simulink model "simulink_problem_2_9_98_14"  (R2014a)
settings: Solver=ode45  SolverMode=SingleTasking  StartTime=0.0  StopTime=10.0  RelTol=1e-3
settings Model: CovMetricSettings=dwe  CovHtmlReporting=off  covSaveCumulativeToWorkspaceVar=off  CovSaveSingleToWorkspaceVar=off  CovExternalEMLEnable=on  CovSFcnEnable=on  Creator=ghost  LastModifiedBy=ghost
settings DataIOCC: LimitDataPoints=off  SaveFormat=StructureWithTime
settings DebuggingCC: MergeDetectMultiDrivingBlocksExec=error  SolverPrmCheckMsg=none  FrameProcessingCompatibilityMsg=error  SFUnexpectedBacktrackingDiag=error  SFNoUnconditionalDefaultTransitionDiag=error
settings HardwareCC: ProdBitPerPointer=64  ProdLargestAtomicFloat=Float  ProdIntDivRoundTo=Zero  ProdEndianess=LittleEndian  ProdHWDeviceType=Specified
settings ModelReferenceCC: PropagateSignalLabelsOutOfModel=on
settings GRTTargetCC: TargetLangStandard=C99 (ISO)  GeneratePreprocessorConditionals=Use local settings

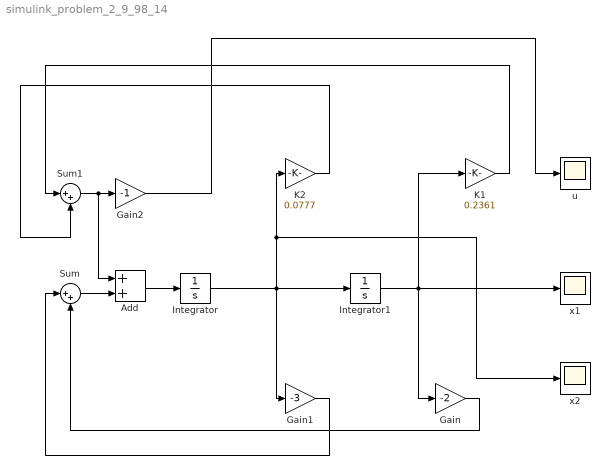
== system simulink_problem_2_9_98_14 ==
  Add : Sum
  Gain : Gain  Gain=-2
  Gain1 : Gain  Gain=-3
  Gain2 : Gain  Gain=-1
  Integrator : Integrator  InitialCondition=2
  Integrator1 : Integrator  InitialCondition=3
  K1 : Gain  Gain=0.2361
  K2 : Gain  Gain=0.0777
  Sum : Sum  Inputs=|++
  Sum1 : Sum  Inputs=|++
  u : Scope
      settings: TimeRange=auto  MaxDataPoints=5000  SaveToWorkspace=off  SaveName=ScopeData2  YMin=-0.97163  YMax=0.10771  SampleTime=-1
  x1 : Scope
      settings: TimeRange=auto  MaxDataPoints=5000  SaveToWorkspace=off  SaveName=ScopeData  YMin=-0.40044  YMax=3.61742  SampleTime=-1
  x2 : Scope
      settings: TimeRange=auto  MaxDataPoints=5000  SaveToWorkspace=off  YMin=-1.90524  YMax=2.43392  SampleTime=-1
  wires:
  Integrator/1 -> K2/1, x2/1, Gain1/1, Integrator1/1
  Integrator1/1 -> K1/1, Gain/1, x1/1
  Gain/1 -> Sum/2
  Gain1/1 -> Sum/1
  K2/1 -> Sum1/2
  K1/1 -> Sum1/1
  Sum/1 -> Add/2
  Add/1 -> Integrator/1
  Sum1/1 -> Gain2/1, Add/1
  Gain2/1 -> u/1
